simulink model "Prova_matrice"  (R2015a)
settings: Solver=ode45  StartTime=0.0  StopTime=10.0  RelTol=1e-3
undefined symbols (not defined in the file or in its folder): B0, B1, B2, B3, m_servo, q_servo, ServoMotor_Gain, tau, x1
settings Model: Creator=Claudio  LastModifiedBy=Claudio

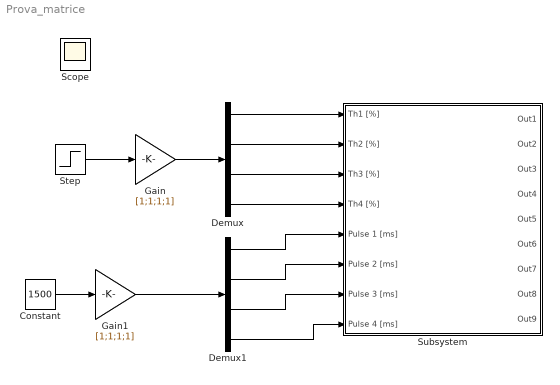
== system Prova_matrice ==
  Constant : Constant  Value=1500
  Demux : Demux
  Demux1 : Demux
  Gain : Gain  Gain=[1;1;1;1]
  Gain1 : Gain  Gain=[1;1;1;1]
  Step : Step  After=50  SampleTime=0
  Subsystem : Subsystem
  Scope : Scope
  wires:
  Step/1 -> Gain/1
  Gain/1 -> Demux/1
  Demux/1 -> Subsystem/1(Th1 [%])
  Demux/2 -> Subsystem/2(Th2 [%])
  Demux/3 -> Subsystem/3(Th3 [%])
  Demux/4 -> Subsystem/4(Th4 [%])
  Constant/1 -> Gain1/1
  Gain1/1 -> Demux1/1
  Demux1/1 -> Subsystem/5(Pulse 1 [ms])
  Demux1/2 -> Subsystem/6(Pulse 2 [ms])
  Demux1/3 -> Subsystem/7(Pulse 3 [ms])
  Demux1/4 -> Subsystem/8(Pulse 4 [ms])

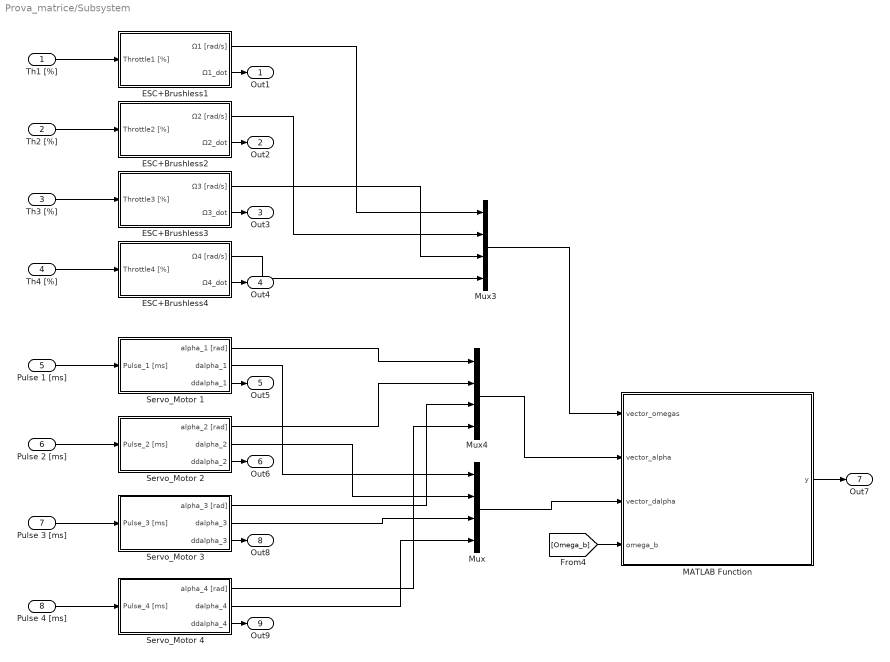
== system Prova_matrice/Subsystem ==
  Th1 [%] : Inport
  Th2 [%] : Inport  Port=2
  Th3 [%] : Inport  Port=3
  Th4 [%] : Inport  Port=4
  Pulse 1 [ms] : Inport  Port=5
  Pulse 2 [ms] : Inport  Port=6
  Pulse 3 [ms] : Inport  Port=7
  Pulse 4 [ms] : Inport  Port=8
  ESC+Brushless1 : Subsystem
  ESC+Brushless2 : Subsystem
  ESC+Brushless3 : Subsystem
  ESC+Brushless4 : Subsystem
  MATLAB Function : MATLAB Function  TreatAsAtomicUnit=on
  Mux : Mux
  Mux3 : Mux
  Mux4 : Mux
  Servo_Motor 1 : Subsystem
  Servo_Motor 2 : Subsystem
  Servo_Motor 3 : Subsystem
  Servo_Motor 4 : Subsystem
  Out1 : Outport
  Out2 : Outport  Port=2
  Out3 : Outport  Port=3
  Out4 : Outport  Port=4
  Out5 : Outport  Port=5
  Out6 : Outport  Port=6
  Out7 : Outport  Port=7
  Out8 : Outport  Port=8
  Out9 : Outport  Port=9
  wires:
  Th1 [%]/1 -> ESC+Brushless1/1(Throttle1 [%])
  Servo_Motor 1/2(dalpha_1) -> Mux/1
  Servo_Motor 2/2(dalpha_2) -> Mux/2
  Pulse 1 [ms]/1 -> Servo_Motor 1/1(Pulse_1 [ms])
  ESC+Brushless1/1(Ω1 [rad/s]) -> Mux3/1
  Th2 [%]/1 -> ESC+Brushless2/1(Throttle2 [%])
  Servo_Motor 3/2(dalpha_3) -> Mux/3
  ESC+Brushless4/1(Ω4 [rad/s]) -> Mux3/4
  [Omega_b] -> MATLAB Function/4(omega_b)
  Pulse 2 [ms]/1 -> Servo_Motor 2/1(Pulse_2 [ms])
  Th4 [%]/1 -> ESC+Brushless4/1(Throttle4 [%])
  Th3 [%]/1 -> ESC+Brushless3/1(Throttle3 [%])
  Pulse 3 [ms]/1 -> Servo_Motor 3/1(Pulse_3 [ms])
  Pulse 4 [ms]/1 -> Servo_Motor 4/1(Pulse_4 [ms])
  Servo_Motor 4/2(dalpha_4) -> Mux/4
  ESC+Brushless2/1(Ω2 [rad/s]) -> Mux3/2
  ESC+Brushless3/1(Ω3 [rad/s]) -> Mux3/3
  Mux3/1 -> MATLAB Function/1(vector_omegas)
  Mux/1 -> MATLAB Function/3(vector_dalpha)
  Servo_Motor 1/1(alpha_1 [rad]) -> Mux4/1
  Servo_Motor 2/1(alpha_2 [rad]) -> Mux4/2
  Servo_Motor 3/1(alpha_3 [rad]) -> Mux4/3
  Servo_Motor 4/1(alpha_4 [rad]) -> Mux4/4
  Mux4/1 -> MATLAB Function/2(vector_alpha)
  ESC+Brushless3/2(Ω3_dot) -> Out3/1
  ESC+Brushless4/2("Ω4_dot ") -> Out4/1
  ESC+Brushless1/2(Ω1_dot) -> Out1/1
  Servo_Motor 1/3(ddalpha_1) -> Out5/1
  Servo_Motor 2/3(ddalpha_2) -> Out6/1
  ESC+Brushless2/2(Ω2_dot) -> Out2/1
  Servo_Motor 3/3(ddalpha_3) -> Out8/1
  Servo_Motor 4/3(ddalpha_4) -> Out9/1
  MATLAB Function/1(y) -> Out7/1

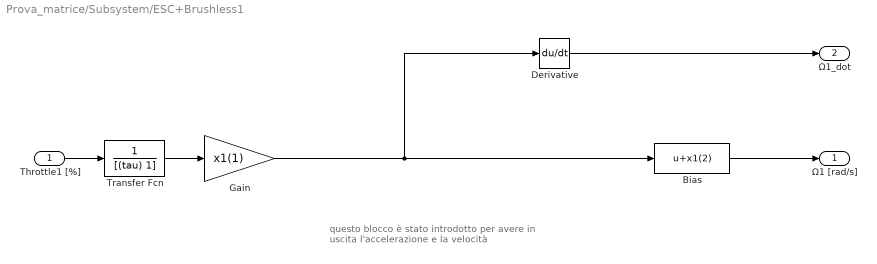
== system Prova_matrice/Subsystem/ESC+Brushless1 ==
  note: questo blocco è stato introdotto per avere in
      | uscita l'accelerazione e la velocità
  Throttle1 [%] : Inport
  Bias : Bias  Bias=x1(2)
  Derivative : Derivative
  Gain : Gain  Gain=x1(1)
  Transfer Fcn : TransferFcn  Denominator=[(tau) 1]
  Ω1 [rad/s] : Outport
  Ω1_dot : Outport  Port=2
  wires:
  Bias/1 -> Ω1 [rad/s]/1
  Throttle1 [%]/1 -> Transfer Fcn/1
  Transfer Fcn/1 -> Gain/1
  Gain/1 -> Bias/1, Derivative/1
  Derivative/1 -> Ω1_dot/1

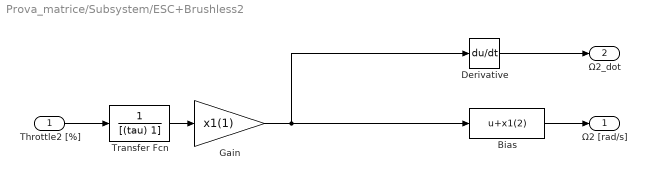
== system Prova_matrice/Subsystem/ESC+Brushless2 ==
  Throttle2 [%] : Inport
  Bias : Bias  Bias=x1(2)
  Derivative : Derivative
  Gain : Gain  Gain=x1(1)
  Transfer Fcn : TransferFcn  Denominator=[(tau) 1]
  Ω2 [rad/s] : Outport
  Ω2_dot : Outport  Port=2
  wires:
  Bias/1 -> Ω2 [rad/s]/1
  Throttle2 [%]/1 -> Transfer Fcn/1
  Transfer Fcn/1 -> Gain/1
  Gain/1 -> Derivative/1, Bias/1
  Derivative/1 -> Ω2_dot/1

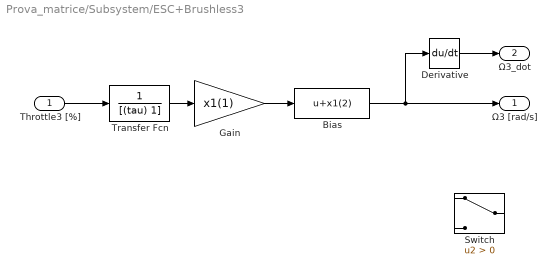
== system Prova_matrice/Subsystem/ESC+Brushless3 ==
  Throttle3 [%] : Inport
  Bias : Bias  Bias=x1(2)
  Derivative : Derivative
  Gain : Gain  Gain=x1(1)
  Switch : Switch  Criteria=u2 > Threshold
  Transfer Fcn : TransferFcn  Denominator=[(tau) 1]
  Ω3 [rad/s] : Outport
  Ω3_dot : Outport  Port=2
  wires:
  Gain/1 -> Bias/1
  Bias/1 -> Derivative/1, Ω3 [rad/s]/1
  Throttle3 [%]/1 -> Transfer Fcn/1
  Transfer Fcn/1 -> Gain/1
  Derivative/1 -> Ω3_dot/1

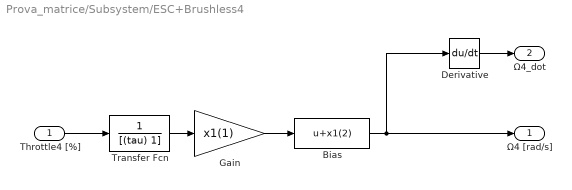
== system Prova_matrice/Subsystem/ESC+Brushless4 ==
  Throttle4 [%] : Inport
  Bias : Bias  Bias=x1(2)
  Derivative : Derivative
  Gain : Gain  Gain=x1(1)
  Transfer Fcn : TransferFcn  Denominator=[(tau) 1]
  Ω4 [rad/s] : Outport
  "Ω4_dot " : Outport  Port=2
  wires:
  Gain/1 -> Bias/1
  Throttle4 [%]/1 -> Transfer Fcn/1
  Transfer Fcn/1 -> Gain/1
  Derivative/1 -> "Ω4_dot "/1
  Bias/1 -> Derivative/1, Ω4 [rad/s]/1

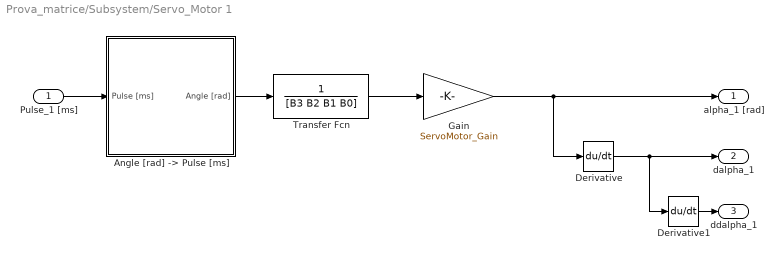
== system Prova_matrice/Subsystem/Servo_Motor 1 ==
  Pulse_1 [ms] : Inport
  "Angle [rad] -> Pulse [ms]" : Subsystem
  Derivative : Derivative
  Derivative1 : Derivative
  Gain : Gain  Gain=ServoMotor_Gain
  Transfer Fcn : TransferFcn  Denominator=[B3 B2 B1 B0]
  alpha_1 [rad] : Outport
  dalpha_1 : Outport  Port=2
  ddalpha_1 : Outport  Port=3
  wires:
  Gain/1 -> Derivative/1, alpha_1 [rad]/1
  Transfer Fcn/1 -> Gain/1
  "Angle [rad] -> Pulse [ms]"/1(Angle [rad]) -> Transfer Fcn/1
  Pulse_1 [ms]/1 -> "Angle [rad] -> Pulse [ms]"/1(Pulse [ms])
  Derivative/1 -> dalpha_1/1, Derivative1/1
  Derivative1/1 -> ddalpha_1/1

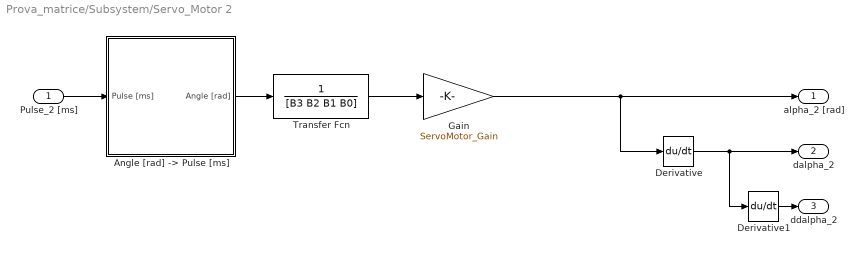
== system Prova_matrice/Subsystem/Servo_Motor 2 ==
  Pulse_2 [ms] : Inport
  "Angle [rad] -> Pulse [ms]" : Subsystem
  Derivative : Derivative
  Derivative1 : Derivative
  Gain : Gain  Gain=ServoMotor_Gain
  Transfer Fcn : TransferFcn  Denominator=[B3 B2 B1 B0]
  alpha_2 [rad] : Outport
  dalpha_2 : Outport  Port=2
  ddalpha_2 : Outport  Port=3
  wires:
  Gain/1 -> Derivative/1, alpha_2 [rad]/1
  Transfer Fcn/1 -> Gain/1
  "Angle [rad] -> Pulse [ms]"/1(Angle [rad]) -> Transfer Fcn/1
  Pulse_2 [ms]/1 -> "Angle [rad] -> Pulse [ms]"/1(Pulse [ms])
  Derivative/1 -> dalpha_2/1, Derivative1/1
  Derivative1/1 -> ddalpha_2/1

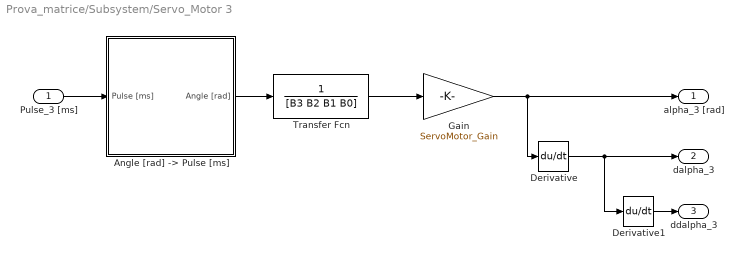
== system Prova_matrice/Subsystem/Servo_Motor 3 ==
  Pulse_3 [ms] : Inport
  "Angle [rad] -> Pulse [ms]" : Subsystem
  Derivative : Derivative
  Derivative1 : Derivative
  Gain : Gain  Gain=ServoMotor_Gain
  Transfer Fcn : TransferFcn  Denominator=[B3 B2 B1 B0]
  alpha_3 [rad] : Outport
  dalpha_3 : Outport  Port=2
  ddalpha_3 : Outport  Port=3
  wires:
  Gain/1 -> Derivative/1, alpha_3 [rad]/1
  Transfer Fcn/1 -> Gain/1
  "Angle [rad] -> Pulse [ms]"/1(Angle [rad]) -> Transfer Fcn/1
  Pulse_3 [ms]/1 -> "Angle [rad] -> Pulse [ms]"/1(Pulse [ms])
  Derivative/1 -> dalpha_3/1, Derivative1/1
  Derivative1/1 -> ddalpha_3/1

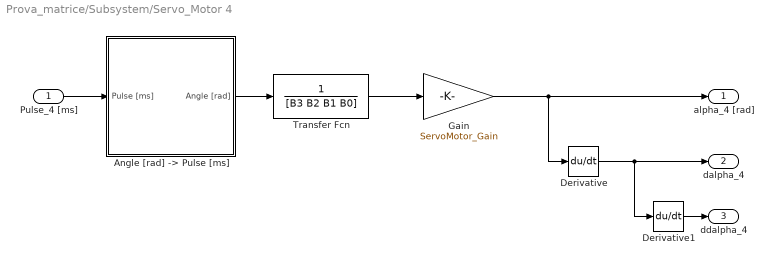
== system Prova_matrice/Subsystem/Servo_Motor 4 ==
  Pulse_4 [ms] : Inport
  "Angle [rad] -> Pulse [ms]" : Subsystem
  Derivative : Derivative
  Derivative1 : Derivative
  Gain : Gain  Gain=ServoMotor_Gain
  Transfer Fcn : TransferFcn  Denominator=[B3 B2 B1 B0]
  alpha_4 [rad] : Outport
  dalpha_4 : Outport  Port=2
  ddalpha_4 : Outport  Port=3
  wires:
  Gain/1 -> Derivative/1, alpha_4 [rad]/1
  Transfer Fcn/1 -> Gain/1
  "Angle [rad] -> Pulse [ms]"/1(Angle [rad]) -> Transfer Fcn/1
  Pulse_4 [ms]/1 -> "Angle [rad] -> Pulse [ms]"/1(Pulse [ms])
  Derivative1/1 -> ddalpha_4/1
  Derivative/1 -> Derivative1/1, dalpha_4/1

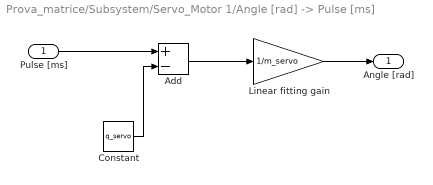
== system Prova_matrice/Subsystem/Servo_Motor 1/Angle [rad] -> Pulse [ms] ==
  Pulse [ms] : Inport
  Add : Sum  Inputs=+-
  Constant : Constant  Value=q_servo
  Linear fitting gain : Gain  Gain=1/m_servo
  Angle [rad] : Outport
  wires:
  Constant/1 -> Add/2
  Add/1 -> Linear fitting gain/1
  Pulse [ms]/1 -> Add/1
  Linear fitting gain/1 -> Angle [rad]/1

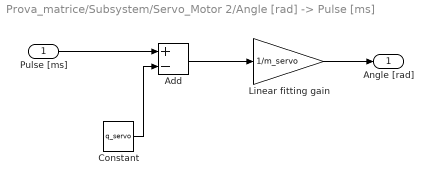
== system Prova_matrice/Subsystem/Servo_Motor 2/Angle [rad] -> Pulse [ms] ==
  Pulse [ms] : Inport
  Add : Sum  Inputs=+-
  Constant : Constant  Value=q_servo
  Linear fitting gain : Gain  Gain=1/m_servo
  Angle [rad] : Outport
  wires:
  Constant/1 -> Add/2
  Add/1 -> Linear fitting gain/1
  Pulse [ms]/1 -> Add/1
  Linear fitting gain/1 -> Angle [rad]/1

== system Prova_matrice/Subsystem/Servo_Motor 3/Angle [rad] -> Pulse [ms] ==
  Pulse [ms] : Inport
  Add : Sum  Inputs=+-
  Constant : Constant  Value=q_servo
  Linear fitting gain : Gain  Gain=1/m_servo
  Angle [rad] : Outport
  wires:
  Constant/1 -> Add/2
  Add/1 -> Linear fitting gain/1
  Pulse [ms]/1 -> Add/1
  Linear fitting gain/1 -> Angle [rad]/1

== system Prova_matrice/Subsystem/Servo_Motor 4/Angle [rad] -> Pulse [ms] ==
  Pulse [ms] : Inport
  Add : Sum  Inputs=+-
  Constant : Constant  Value=q_servo
  Linear fitting gain : Gain  Gain=1/m_servo
  Angle [rad] : Outport
  wires:
  Constant/1 -> Add/2
  Add/1 -> Linear fitting gain/1
  Pulse [ms]/1 -> Add/1
  Linear fitting gain/1 -> Angle [rad]/1

== matlab function Prova_matrice/Subsystem/MATLAB Function ==
  data: vector_omegas input; vector_alpha input; vector_dalpha input; y output; omega_b input
function y = fcn(vector_omegas,vector_alpha,vector_dalpha,omega_b)
%#codegen

% Rotation matrix from Body to propeller group
omega_pi = [0;0;0;0];
        
 for i=1:length(vector_omegas)
     psi = (i-1)*pi/2;
     phi = vector_alpha(1)
     R_PiB = [cos(psi),           sin(psi),        0;
       -cos(phi)*sin(psi),  cos(phi)*cos(psi), sin(phi);
        sin(phi)*sin(psi), -cos(psi)*sin(phi), cos(phi)];
     omega_pi(i) = R_PiB*omega_b+ [vector_dalpha(i);0;vector_domegas(i)]';
 end
 result = omega_pi;

y = result;
